simulink model "Lab1_DynamicDecoupledPlantModel"  (R2019a)
settings: Solver=VariableStepAuto  StartTime=0.0  StopTime=100  RelTol=1e-3
libraries: cstblocks x2
settings Model: Creator=emma  LastModifiedBy=emma

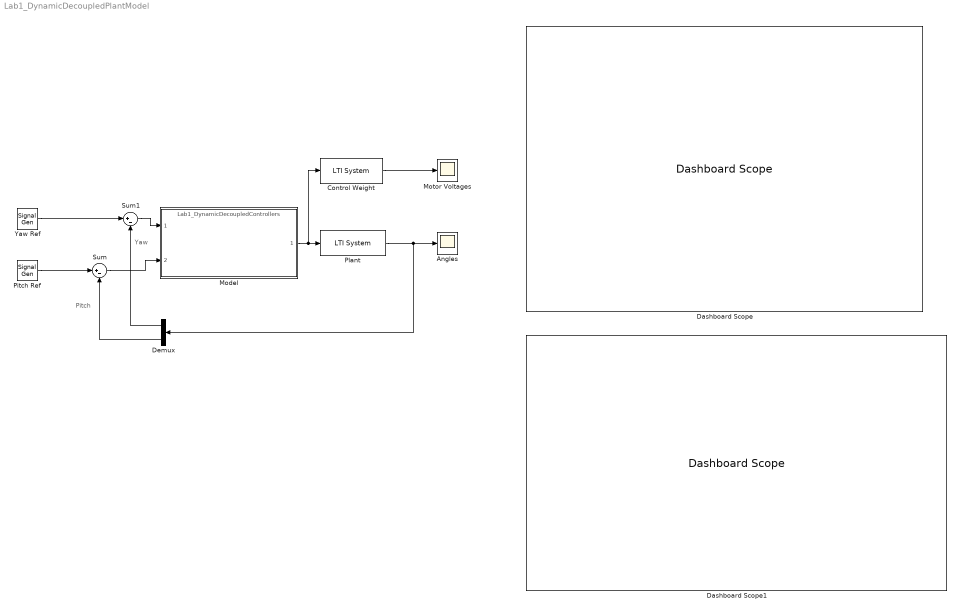
== system Lab1_DynamicDecoupledPlantModel ==
  note: Yaw
  note: Pitch
  Angles : Scope
  Control Weight : cstblocks/LTI System  sys=Wu  IC=[]
  Dashboard Scope : DashboardScope
  Dashboard Scope1 : DashboardScope
  Demux : Demux  Outputs=2
  Model : ModelReference  ModelNameDialog=Lab1_DynamicDecoupledControllers.slx  SimulationMode=Normal  ModelReferenceVersion=1.3
  Motor Voltages : Scope
  Pitch Ref : SignalGenerator  WaveForm=square  Amplitude=pi/6  Frequency=0.4  Units=rad/sec
  Plant : cstblocks/LTI System  sys=Gnom  IC=[]
  Sum : Sum  Inputs=|+-
  Sum1 : Sum  Inputs=|+-
  Yaw Ref : SignalGenerator  WaveForm=square  Amplitude=pi/4  Frequency=0.5  Units=rad/sec
  wires:
  Yaw Ref/1 -> Sum1/1
  Control Weight/1 -> Motor Voltages/1
  Plant/1 -> Demux/1, Angles/1
  Pitch Ref/1 -> Sum/1
  Demux/1 -> Sum1/2
  Demux/2 -> Sum/2
  Model/1 -> Control Weight/1, Plant/1
  Sum1/1 -> Model/1
  Sum/1 -> Model/2
